simulink model "comp_debounce"  (R2014a)
settings: Solver=FixedStepDiscrete  StartTime=0.0  StopTime=10.0  RelTol=1e-3
libraries: simulink x2, hdlsllib x1
settings Model: Creator=User  LastModifiedBy=User
settings OptimizationCC: InlineParams=on

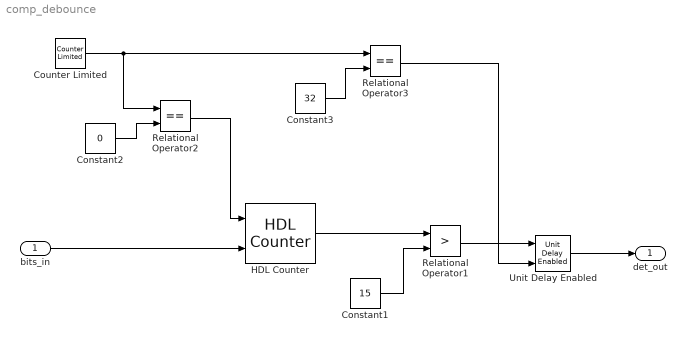
== system comp_debounce ==
  bits_in : Inport  OutDataTypeStr=boolean
  Constant1 : Constant  Value=15  OutDataTypeStr=Inherit: Inherit via back propagation
  Constant2 : Constant  Value=0  OutDataTypeStr=Inherit: Inherit via back propagation
  Constant3 : Constant  Value=32  OutDataTypeStr=Inherit: Inherit via back propagation
  Counter Limited : simulink/Sources/Counter Limited  uplimit=32  tsamp=-1
  HDL Counter : hdlsllib/HDL Operations/HDL Counter  CountType=Free running  CountInit=0  CountStep=1  CountMax=128  CountFromType=Initial value  CountFrom=0  CountResetPort=on  CountLoadPort=off  CountEnbPort=on  CountDirPort=off  CountDataType=Unsigned  CountWordLen=8  CountFracLen=0  CountSampTime=1
  Relational Operator1 : RelationalOperator  Operator=>  OutDataTypeStr=boolean
  Relational Operator2 : RelationalOperator  Operator===  OutDataTypeStr=boolean
  Relational Operator3 : RelationalOperator  Operator===  OutDataTypeStr=boolean
  Unit Delay Enabled : simulink/Additional Math & Discrete/Additional Discrete/Unit Delay Enabled  vinit=600  tsamp=-1
  det_out : Outport  OutDataTypeStr=boolean
  wires:
  HDL Counter/1 -> Relational Operator1/1
  Constant1/1 -> Relational Operator1/2
  Unit Delay Enabled/1 -> det_out/1
  Counter Limited/1 -> Relational Operator2/1, Relational Operator3/1
  Constant2/1 -> Relational Operator2/2
  Constant3/1 -> Relational Operator3/2
  Relational Operator3/1 -> Unit Delay Enabled/2
  Relational Operator2/1 -> HDL Counter/1
  bits_in/1 -> HDL Counter/2
  Relational Operator1/1 -> Unit Delay Enabled/1
